simulink model "LQR_2_corrupted"  (R2025b)
settings: Solver=VariableStepAuto  StartTime=0.0  StopTime=10.0  RelTol=1e-3
undefined symbols (not defined in the file): ic_xy, ic_xz, ic_yz, K_vert, K_xy, params, rate_lim, T_max
settings Model: Creator=JPham  LastModifiedBy=JPham

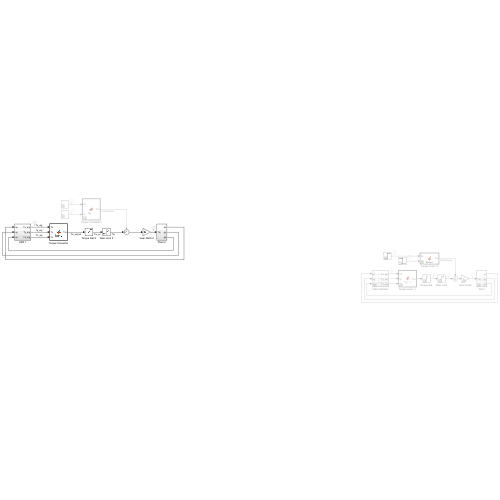
[thumbnail: Simulink's stored preview of the top-level diagram]
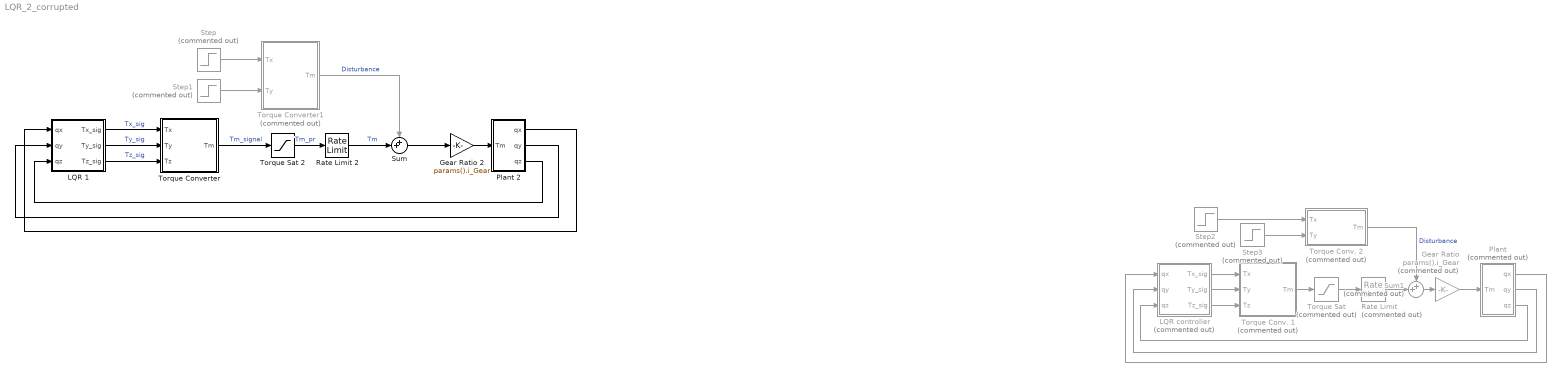
== system LQR_2_corrupted ==
  Gear Ratio : Gain  Commented=on  Gain=params().i_Gear
  Gear Ratio 2 : Gain  Gain=params().i_Gear
  LQR 1 : Subsystem
  LQR controller : Subsystem  Commented=on
  Plant : Subsystem  Commented=on
  Plant 2 : Subsystem
  Rate Limit : RateLimiter  Commented=on  RisingSlewLimit=rate_lim  FallingSlewLimit=-rate_lim  SampleTimeMode=inherited
  Rate Limit 2 : RateLimiter  RisingSlewLimit=rate_lim  FallingSlewLimit=-rate_lim  SampleTimeMode=inherited
  Step : Step  Commented=on  Time=2  After=2  SampleTime=0
  Step1 : Step  Commented=on  Time=2  After=-2  SampleTime=0
  Step2 : Step  Commented=on  Time=2  After=2  SampleTime=0
  Step3 : Step  Commented=on  Time=2  After=-2  SampleTime=0
  Sum : Sum  Inputs=++|
  Sum1 : Sum  Commented=on  Inputs=++|
  Torque Conv. 1 : MATLAB Function  Commented=on  TreatAsAtomicUnit=on
  Torque Conv. 2 : MATLAB Function  Commented=on  TreatAsAtomicUnit=on
  Torque Converter : MATLAB Function  TreatAsAtomicUnit=on
  Torque Converter1 : MATLAB Function  Commented=on  TreatAsAtomicUnit=on
  Torque Sat : Saturate  Commented=on  UpperLimit=T_max  LowerLimit=-T_max
  Torque Sat 2 : Saturate  UpperLimit=T_max  LowerLimit=-T_max
  wires:
  Torque Converter/1(Tm) -> Torque Sat 2/1  "Tm_signal"
  LQR 1/1(Tx_sig) -> Torque Converter/1(Tx)  "Tx_sig"
  LQR 1/2(Ty_sig) -> Torque Converter/2(Ty)  "Ty_sig"
  LQR 1/3(Tz_sig) -> Torque Converter/3(Tz)  "Tz_sig"
  Plant 2/2(qy) -> LQR 1/2(qy)
  Plant 2/1(qx) -> LQR 1/1(qx)
  Plant 2/3(qz) -> LQR 1/3(qz)
  Step/1 -> Torque Converter1/1(Tx)
  Step1/1 -> Torque Converter1/2(Ty)
  Gear Ratio 2/1 -> Plant 2/1(Tm)
  Torque Converter1/1(Tm) -> Sum/1  "Disturbance"
  Torque Sat 2/1 -> Rate Limit 2/1  "Tm_pr"
  Rate Limit 2/1 -> Sum/2  "Tm"
  Sum/1 -> Gear Ratio 2/1
  Plant/1(qx) -> LQR controller/1(qx)
  LQR controller/1(Tx_sig) -> Torque Conv. 1/1(Tx)
  Plant/3(qz) -> LQR controller/3(qz)
  Sum1/1 -> Gear Ratio/1
  LQR controller/2(Ty_sig) -> Torque Conv. 1/2(Ty)
  Step2/1 -> Torque Conv. 2/1(Tx)
  Gear Ratio/1 -> Plant/1(Tm)
  Step3/1 -> Torque Conv. 2/2(Ty)
  LQR controller/3(Tz_sig) -> Torque Conv. 1/3(Tz)
  Plant/2(qy) -> LQR controller/2(qy)
  Torque Sat/1 -> Rate Limit/1
  Torque Conv. 2/1(Tm) -> Sum1/1  "Disturbance"
  Rate Limit/1 -> Sum1/2
  Torque Conv. 1/1(Tm) -> Torque Sat/1

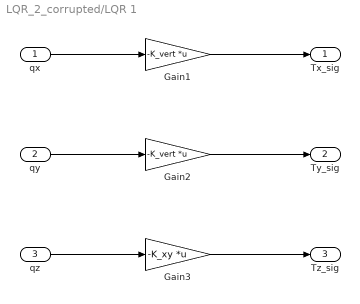
== system LQR_2_corrupted/LQR 1 ==
  qx : Inport
  qy : Inport  Port=2
  qz : Inport  Port=3
  Gain1 : Gain  Gain=-K_vert  Multiplication=Matrix(K*u) (u vector)
  Gain2 : Gain  Gain=-K_vert  Multiplication=Matrix(K*u) (u vector)
  Gain3 : Gain  Gain=-K_xy  Multiplication=Matrix(K*u) (u vector)
  Tx_sig : Outport
  Ty_sig : Outport  Port=2
  Tz_sig : Outport  Port=3
  wires:
  Gain3/1 -> Tz_sig/1
  qy/1 -> Gain2/1
  Gain1/1 -> Tx_sig/1
  Gain2/1 -> Ty_sig/1
  qz/1 -> Gain3/1
  qx/1 -> Gain1/1

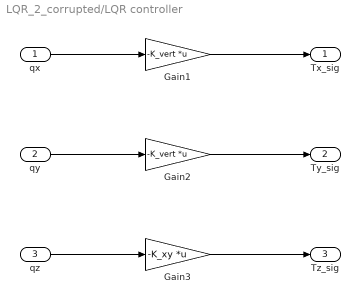
== system LQR_2_corrupted/LQR controller ==
  qx : Inport
  qy : Inport  Port=2
  qz : Inport  Port=3
  Gain1 : Gain  Gain=-K_vert  Multiplication=Matrix(K*u) (u vector)
  Gain2 : Gain  Gain=-K_vert  Multiplication=Matrix(K*u) (u vector)
  Gain3 : Gain  Gain=-K_xy  Multiplication=Matrix(K*u) (u vector)
  Tx_sig : Outport
  Ty_sig : Outport  Port=2
  Tz_sig : Outport  Port=3
  wires:
  Gain3/1 -> Tz_sig/1
  qy/1 -> Gain2/1
  Gain1/1 -> Tx_sig/1
  Gain2/1 -> Ty_sig/1
  qz/1 -> Gain3/1
  qx/1 -> Gain1/1

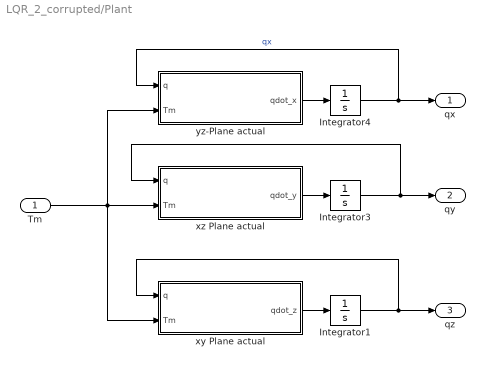
== system LQR_2_corrupted/Plant ==
  Tm : Inport
  Integrator1 : Integrator  InitialCondition=ic_xy
  Integrator3 : Integrator  InitialCondition=ic_xz  ContinuousStateAttributes='angle'
  Integrator4 : Integrator  InitialCondition=ic_yz  ContinuousStateAttributes='angle'
  xy Plane actual : MATLAB Function  TreatAsAtomicUnit=on
  xz Plane actual : MATLAB Function  TreatAsAtomicUnit=on
  yz-Plane actual : MATLAB Function  TreatAsAtomicUnit=on
  qx : Outport
  qy : Outport  Port=2
  qz : Outport  Port=3
  wires:
  Integrator1/1 -> xy Plane actual/1(q), qz/1
  Tm/1 -> xy Plane actual/2(Tm), yz-Plane actual/2(Tm), xz Plane actual/2(Tm)
  xz Plane actual/1(qdot_y) -> Integrator3/1
  yz-Plane actual/1(qdot_x) -> Integrator4/1
  xy Plane actual/1(qdot_z) -> Integrator1/1
  Integrator4/1 -> yz-Plane actual/1(q), qx/1  "qx"
  Integrator3/1 -> xz Plane actual/1(q), qy/1

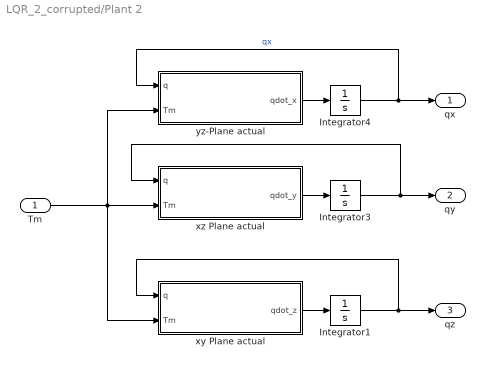
== system LQR_2_corrupted/Plant 2 ==
  Tm : Inport
  Integrator1 : Integrator  InitialCondition=ic_xy
  Integrator3 : Integrator  InitialCondition=ic_xz  ContinuousStateAttributes='angle'
  Integrator4 : Integrator  InitialCondition=ic_yz  ContinuousStateAttributes='angle'
  xy Plane actual : MATLAB Function  TreatAsAtomicUnit=on
  xz Plane actual : MATLAB Function  TreatAsAtomicUnit=on
  yz-Plane actual : MATLAB Function  TreatAsAtomicUnit=on
  qx : Outport
  qy : Outport  Port=2
  qz : Outport  Port=3
  wires:
  Integrator1/1 -> xy Plane actual/1(q), qz/1
  Tm/1 -> xy Plane actual/2(Tm), yz-Plane actual/2(Tm), xz Plane actual/2(Tm)
  xz Plane actual/1(qdot_y) -> Integrator3/1
  yz-Plane actual/1(qdot_x) -> Integrator4/1
  xy Plane actual/1(qdot_z) -> Integrator1/1
  Integrator4/1 -> yz-Plane actual/1(q), qx/1  "qx"
  Integrator3/1 -> xz Plane actual/1(q), qy/1

== matlab function LQR_2_corrupted/Plant/xy Plane actual ==
  data: q input; Tm input; qdot_z output
function qdot_z = f(q, Tm)
    % Define dimensions for code generation
    % x is 2x1 state: [theta; theta_dot]
    % Tm is the torques from 3 motors
    % p is the parameter structure
    
    theta   = q(1); % theta
    dottheta= q(2); % theta_dot
    alpha = params().alpha;
    beta  = params().beta;
    Tz = Tm(1) + Tm(2) + Tm(3);

    p = params;
    
    T_f = ((p.r_ball*p.r_omni*p.Theta_body_xy*sin(p.alpha))...
        /((p.r_omni)^2*p.Theta_body_xy+(p.r_ball)^2*p.Theta_virt_xy*(sin(p.alpha))^2))*Tz;

    ddottheta = -(p.r_ball*sin(p.alpha))*(p.r_ball*p.Theta_virt_xy*sin(p.alpha)+p.r_omni*p.Theta_ball)*T_f...
        /((p.r_omni)^2*p.Theta_body_xy*p.Theta_ball+(p.r_ball)^2*(p.Theta_body_xy+p.Theta_ball)*p.Theta_virt_xy*(sin(p.alpha))^2);
    
    % Assemble qdot_z
    qdot_z = [dottheta;
                ddottheta];
end

== matlab function LQR_2_corrupted/Torque Converter1 ==
  data: Tx input; Ty input; Tm output
function Tm = Tconv(Tx, Ty)
    Tz=0;
    alpha = params().alpha;
    beta  = params().beta;
    % Omni to motors torque convert matrix
    T_o2m = (1/(3*cos(alpha)))*...
    [2*cos(beta)                  , -2*sin(beta)                , cos(alpha);
    (-sqrt(3)*sin(beta)-cos(beta)), (sin(beta)-sqrt(3)*cos(beta)), cos(alpha);
     (sqrt(3)*sin(beta)-cos(beta)), (sin(beta)+sqrt(3)*cos(beta)), cos(alpha)
    ];
    Tm = T_o2m*[Tx; Ty; Tz];
    Tm = Tm./params().i_Gear;
end

== matlab function LQR_2_corrupted/Plant/xz Plane actual ==
  data: q input; Tm input; qdot_y output
function qdot_y = f(q, Tm)
    % Define dimensions for code generation
    % x is 4x1 state: [phi; theta; phi_dot; theta_dot]
    % Tm is the torque from the three motors
    % p is the parameter structure

    % Convert motor torque to omniwheel torque
    alpha = params().alpha;
    beta  = params().beta;
    Ty = cos(alpha)*(-Tm(1)*sin(beta)) - Tm(2)*cos(beta + pi/6) + Tm(3)*cos(beta - pi/6);

    % States
    phi     = q(1); % phi
    theta   = q(2); % theta
    dotphi  = q(3); % phi_dot
    dottheta= q(4); % theta_dot
    
    p = params;
    % Aux Parameters
    m_tot = p.m_ball + p.m_body + p.m_virt;
    r_tot = p.r_ball + p.r_omni;
    gamma = p.l*p.m_body + (p.r_ball + p.r_omni)*p.m_virt;
    
    % M matrix
    M11 = m_tot * p.r_ball^2 + p.Theta_ball + (p.r_ball / p.r_omni)^2 * p.Theta_virt_vertical;
    M12 = -(p.r_ball / p.r_omni^2) * r_tot * p.Theta_virt_vertical + gamma * p.r_ball*cos(theta); 
    M22 = (r_tot^2 / p.r_omni^2) * p.Theta_virt_vertical + p.Theta_body_vertical + ...
           p.m_body * p.l^2 + p.m_virt * r_tot^2;
    M21 = M12;

    M = [M11, M12;
         M21, M22];
    
    % C vector
    Cvec = [ -p.r_ball*gamma*sin(theta)*dottheta^2; 
              0 ];
    % G vector
    Gvec = [ 0; 
            -p.g*sin(theta)*gamma ];
    % S vector (f_NP = S*u(t))
    S = [ p.r_ball / p.r_omni; -p.r_ball / p.r_omni ];
    
    % --- Dynamics Calculation ---
    F_np = S * Ty; 
    
    % Solve for qdd from M * qdd + C + G = F_np
    % qddot = M \ (F_np - C - G) = [theta_doubledot; phi_doubledot]
    qddot = M \ (F_np - Cvec - Gvec);
    
    % Assemble qdot_y
    qdot_y = [dotphi;
              dottheta;
              qddot(1);
              qddot(2)];
end

== matlab function LQR_2_corrupted/Plant/yz-Plane actual ==
  data: q input; Tm input; qdot_x output
function qdot_x = f(q, Tm)
    % Define dimensions for code generation
    % x is 4x1 state: [phi; theta; phi_dot; theta_dot]
    % Tm is the torque from the three motors
    % p is the parameter structure, loaded into simulink in Model Explorer

    % Convert motor torque to omniwheel torque
    alpha = params().alpha;
    beta  = params().beta;
    Tx = cos(alpha)*(Tm(1)*cos(beta)) - Tm(2)*sin(beta + pi/6) + Tm(3)*sin(beta - pi/6);

    % States
    phi     = q(1); % phi
    theta   = q(2); % theta
    dotphi  = q(3); % phi_dot
    dottheta= q(4); % theta_dot
    
    p = params;
    % Aux Parameters
    m_tot = p.m_ball + p.m_body + p.m_virt;
    r_tot = p.r_ball + p.r_omni;
    gamma = p.l*p.m_body + (p.r_ball + p.r_omni)*p.m_virt;
    
    % M matrix
    M11 = m_tot * p.r_ball^2 + p.Theta_ball + (p.r_ball / p.r_omni)^2 * p.Theta_virt_vertical;
    M12 = -(p.r_ball / p.r_omni^2) * r_tot * p.Theta_virt_vertical + gamma * p.r_ball*cos(theta); 
    M22 = (r_tot^2 / p.r_omni^2) * p.Theta_virt_vertical + p.Theta_body_vertical + ...
           p.m_body * p.l^2 + p.m_virt * r_tot^2;
    M21 = M12;

    M = [M11, M12;
         M21, M22];
    
    % C vector
    Cvec = [ -p.r_ball*gamma*sin(theta)*dottheta^2; 
              0 ];
    % G vector
    Gvec = [ 0; 
            -p.g*sin(theta)*gamma ];
    % S vector (f_NP = S*u(t))
    S = [ p.r_ball / p.r_omni; -p.r_ball / p.r_omni ];
    
    % --- Dynamics Calculation ---
    F_np = S * Tx; 
    
    % Solve for qdd from M * qdd + C + G = F_np
    % qddot = M \ (F_np - C - G) = [theta_doubledot; phi_doubledot]
    qddot = M \ (F_np - Cvec - Gvec);
    
    % Assemble qdot_vertical
    qdot_x = [dotphi;
              dottheta;
              qddot(1);
              qddot(2)];
end

== matlab function LQR_2_corrupted/Torque Conv. 1 ==
  data: Tx input; Ty input; Tm output; Tz input
function Tm = Tconv(Tx, Ty, Tz)
    alpha = params().alpha;
    beta  = params().beta;
    % Omni to motors torque convert matrix
    T_o2m = (1/(3*cos(alpha)))*...
    [2*cos(beta)                  , -2*sin(beta)                , cos(alpha);
    (-sqrt(3)*sin(beta)-cos(beta)), (sin(beta)-sqrt(3)*cos(beta)), cos(alpha);
     (sqrt(3)*sin(beta)-cos(beta)), (sin(beta)+sqrt(3)*cos(beta)), cos(alpha)
    ];
    Tm = T_o2m*[Tx; Ty; Tz];
    Tm = Tm./params().i_Gear;
end

== matlab function LQR_2_corrupted/Torque Conv. 2 ==
  data: Tx input; Ty input; Tm output
function Tm = Tconv(Tx, Ty)
    Tz=0;
    alpha = params().alpha;
    beta  = params().beta;
    % Omni to motors torque convert matrix
    T_o2m = (1/(3*cos(alpha)))*...
    [2*cos(beta)                  , -2*sin(beta)                , cos(alpha);
    (-sqrt(3)*sin(beta)-cos(beta)), (sin(beta)-sqrt(3)*cos(beta)), cos(alpha);
     (sqrt(3)*sin(beta)-cos(beta)), (sin(beta)+sqrt(3)*cos(beta)), cos(alpha)
    ];
    Tm = T_o2m*[Tx; Ty; Tz];
    Tm = Tm./params().i_Gear;
end

== matlab function LQR_2_corrupted/Torque Converter ==
  data: Tx input; Ty input; Tm output; Tz input
function Tm = Tconv(Tx, Ty, Tz)
    alpha = params().alpha;
    beta  = params().beta;
    % Omni to motors torque convert matrix
    T_o2m = (1/(3*cos(alpha)))*...
    [2*cos(beta)                  , -2*sin(beta)                , cos(alpha);
    (-sqrt(3)*sin(beta)-cos(beta)), (sin(beta)-sqrt(3)*cos(beta)), cos(alpha);
     (sqrt(3)*sin(beta)-cos(beta)), (sin(beta)+sqrt(3)*cos(beta)), cos(alpha)
    ];
    Tm = T_o2m*[Tx; Ty; Tz];
    Tm = Tm./params().i_Gear;
end

== matlab function LQR_2_corrupted/Plant 2/xy Plane actual ==
  data: q input; Tm input; qdot_z output
function qdot_z = f(q, Tm)
    % Define dimensions for code generation
    % x is 2x1 state: [theta; theta_dot]
    % Tm is the torques from 3 motors
    % p is the parameter structure
    
    theta   = q(1); % theta
    dottheta= q(2); % theta_dot
    alpha = params().alpha;
    beta  = params().beta;
    Tz = Tm(1) + Tm(2) + Tm(3);

    p = params;
    
    T_f = ((p.r_ball*p.r_omni*p.Theta_body_xy*sin(p.alpha))...
        /((p.r_omni)^2*p.Theta_body_xy+(p.r_ball)^2*p.Theta_virt_xy*(sin(p.alpha))^2))*Tz;

    ddottheta = -(p.r_ball*sin(p.alpha))*(p.r_ball*p.Theta_virt_xy*sin(p.alpha)+p.r_omni*p.Theta_ball)*T_f...
        /((p.r_omni)^2*p.Theta_body_xy*p.Theta_ball+(p.r_ball)^2*(p.Theta_body_xy+p.Theta_ball)*p.Theta_virt_xy*(sin(p.alpha))^2);
    
    % Assemble qdot_z
    qdot_z = [dottheta;
                ddottheta];
end

== matlab function LQR_2_corrupted/Plant 2/xz Plane actual ==
  data: q input; Tm input; qdot_y output
function qdot_y = f(q, Tm)
    % Define dimensions for code generation
    % x is 4x1 state: [phi; theta; phi_dot; theta_dot]
    % Tm is the torque from the three motors
    % p is the parameter structure

    % Convert motor torque to omniwheel torque
    alpha = params().alpha;
    beta  = params().beta;
    Ty = cos(alpha)*(-Tm(1)*sin(beta)) - Tm(2)*cos(beta + pi/6) + Tm(3)*cos(beta - pi/6);

    % States
    phi     = q(1); % phi
    theta   = q(2); % theta
    dotphi  = q(3); % phi_dot
    dottheta= q(4); % theta_dot
    
    p = params;
    % Aux Parameters
    m_tot = p.m_ball + p.m_body + p.m_virt;
    r_tot = p.r_ball + p.r_omni;
    gamma = p.l*p.m_body + (p.r_ball + p.r_omni)*p.m_virt;
    
    % M matrix
    M11 = m_tot * p.r_ball^2 + p.Theta_ball + (p.r_ball / p.r_omni)^2 * p.Theta_virt_vertical;
    M12 = -(p.r_ball / p.r_omni^2) * r_tot * p.Theta_virt_vertical + gamma * p.r_ball*cos(theta); 
    M22 = (r_tot^2 / p.r_omni^2) * p.Theta_virt_vertical + p.Theta_body_vertical + ...
           p.m_body * p.l^2 + p.m_virt * r_tot^2;
    M21 = M12;

    M = [M11, M12;
         M21, M22];
    
    % C vector
    Cvec = [ -p.r_ball*gamma*sin(theta)*dottheta^2; 
              0 ];
    % G vector
    Gvec = [ 0; 
            -p.g*sin(theta)*gamma ];
    % S vector (f_NP = S*u(t))
    S = [ p.r_ball / p.r_omni; -p.r_ball / p.r_omni ];
    
    % --- Dynamics Calculation ---
    F_np = S * Ty; 
    
    % Solve for qdd from M * qdd + C + G = F_np
    % qddot = M \ (F_np - C - G) = [theta_doubledot; phi_doubledot]
    qddot = M \ (F_np - Cvec - Gvec);
    
    % Assemble qdot_y
    qdot_y = [dotphi;
              dottheta;
              qddot(1);
              qddot(2)];
end

== matlab function LQR_2_corrupted/Plant 2/yz-Plane actual ==
  data: q input; Tm input; qdot_x output
function qdot_x = f(q, Tm)
    % Define dimensions for code generation
    % x is 4x1 state: [phi; theta; phi_dot; theta_dot]
    % Tm is the torque from the three motors
    % p is the parameter structure, loaded into simulink in Model Explorer

    % Convert motor torque to omniwheel torque
    alpha = params().alpha;
    beta  = params().beta;
    Tx = cos(alpha)*(Tm(1)*cos(beta)) - Tm(2)*sin(beta + pi/6) + Tm(3)*sin(beta - pi/6);

    % States
    phi     = q(1); % phi
    theta   = q(2); % theta
    dotphi  = q(3); % phi_dot
    dottheta= q(4); % theta_dot
    
    p = params;
    % Aux Parameters
    m_tot = p.m_ball + p.m_body + p.m_virt;
    r_tot = p.r_ball + p.r_omni;
    gamma = p.l*p.m_body + (p.r_ball + p.r_omni)*p.m_virt;
    
    % M matrix
    M11 = m_tot * p.r_ball^2 + p.Theta_ball + (p.r_ball / p.r_omni)^2 * p.Theta_virt_vertical;
    M12 = -(p.r_ball / p.r_omni^2) * r_tot * p.Theta_virt_vertical + gamma * p.r_ball*cos(theta); 
    M22 = (r_tot^2 / p.r_omni^2) * p.Theta_virt_vertical + p.Theta_body_vertical + ...
           p.m_body * p.l^2 + p.m_virt * r_tot^2;
    M21 = M12;

    M = [M11, M12;
         M21, M22];
    
    % C vector
    Cvec = [ -p.r_ball*gamma*sin(theta)*dottheta^2; 
              0 ];
    % G vector
    Gvec = [ 0; 
            -p.g*sin(theta)*gamma ];
    % S vector (f_NP = S*u(t))
    S = [ p.r_ball / p.r_omni; -p.r_ball / p.r_omni ];
    
    % --- Dynamics Calculation ---
    F_np = S * Tx; 
    
    % Solve for qdd from M * qdd + C + G = F_np
    % qddot = M \ (F_np - C - G) = [theta_doubledot; phi_doubledot]
    qddot = M \ (F_np - Cvec - Gvec);
    
    % Assemble qdot_vertical
    qdot_x = [dotphi;
              dottheta;
              qddot(1);
              qddot(2)];
end
